simulink model "regulacja_pogodowa_model"  (R2022b)
settings: Solver=VariableStepAuto  StartTime=0.0  StopTime=tmax  MaxStep=0.2  RelTol=1e-3
values from neighbouring files (symbols this model uses):
  ap_wz = (TwpN - TzewN)/(TwewN - TzewN)    (= 3.25)    [obliczenia.m]    (also in obliczenia2.m)
  az_wz = (TwzN - TzewN)/(TwewN - TzewN)    (= 3.75)    [obliczenia.m]    (also in obliczenia2.m)
  bp_wz = (TwpN - TwewN)/(TwewN - TzewN)    (= 2.25)    [obliczenia.m]    (also in obliczenia2.m)
  bz_wz = (TwzN - TwewN)/(TwewN - TzewN)    (= 2.75)    [obliczenia.m]    (also in obliczenia2.m)
  dFmw = 0    [obliczenia.m]    (also in obliczenia2.m)
  Ki = 1    [obliczenia.m]    (also in obliczenia2.m = 0)
  Kp = 0.9*TczasRp2/(kRp2*TopuRp2)    (= 0.110974924224)    [obliczenia.m]    (also in obliczenia2.m = 1.05226274907)
  kRp = (1.3488)/0.02    (= 67.44)    [obliczenia.m]
  kRp2 = (71.1034-70)/0.02    (= 55.17)    [obliczenia.m]
  TczasRp = 10670-2648    (= 8022)    [obliczenia.m]
  TczasRp2 = 20334-TopuRp2    (= 17728)    [obliczenia.m]
  TemVec = [-20:20]    [obliczenia.m]    (also in obliczenia2.m = [-20,20])
  Ti = 3.33*TopuRp2/Kp    (= 78197.6654695)    [obliczenia.m]    (also in obliczenia2.m = 11755.1763626)
  TopN = TgpN    (= 70)    [obliczenia.m]    (also in obliczenia2.m)
  TopuRp = 2648 - 2000    (= 648)    [obliczenia.m]
  TopuRp2 = 4606 - tsok    (= 2606)    [obliczenia.m]
  Toz0 = TozN    (= 90)    [obliczenia.m]    (also in obliczenia2.m)
  TozN = TgzN    (= 90)    [obliczenia.m]    (also in obliczenia2.m)
  tsok = 2000    [obliczenia.m]    (also in obliczenia2.m = 80000)
  TwewN = 20    [obliczenia.m]    (also in obliczenia2.m)
undefined symbols (not defined in the file or in its folder): dToz
settings Model: Creator=asialalala  LastModifiedBy=asialalala
settings DataIOCC: ReturnWorkspaceOutputs=off

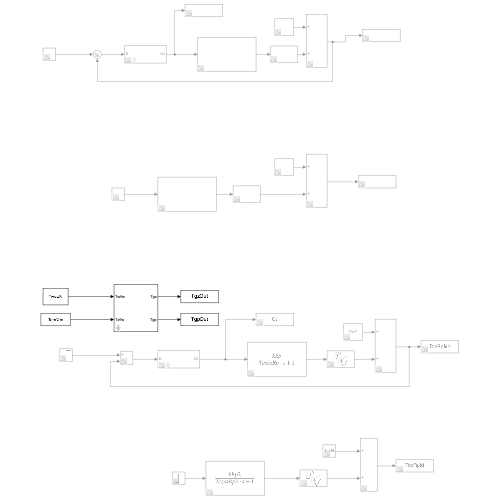
[thumbnail: Simulink's stored preview of the top-level diagram]
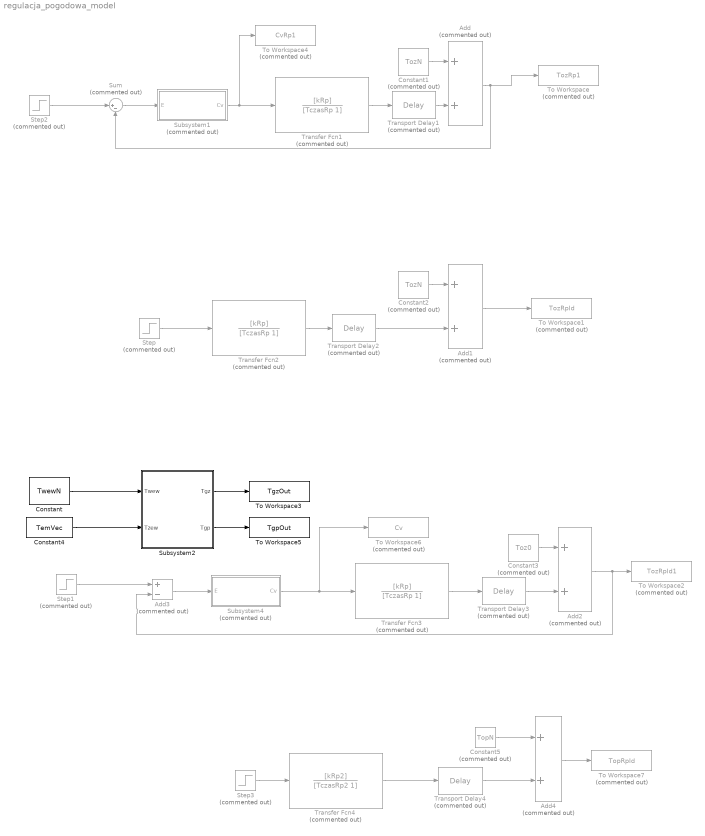
== system regulacja_pogodowa_model ==
  Add{,1..2,4} (4 alike) : Sum  Commented=on
  Add3 : Sum  Commented=on  Inputs=+-
  Constant : Constant  Value=TwewN
  Constant1 : Constant  Commented=on  Value=TozN
  Constant2 : Constant  Commented=on  Value=TozN
  Constant3 : Constant  Commented=on  Value=Toz0
  Constant4 : Constant  Value=TemVec
  Constant5 : Constant  Commented=on  Value=TopN
  Step : Step  Commented=on  Time=tsok  After=dFmw  SampleTime=0
  Step1 : Step  Commented=on  Time=tsok  Before=Toz0  After=Toz0+1  SampleTime=0
  Step2 : Step  Commented=on  Time=tsok  Before=TozN  After="TozN  + dToz"  SampleTime=0
  Step3 : Step  Commented=on  Time=tsok  After=dFmw  SampleTime=0
  Subsystem1 : Subsystem  Commented=on  mask{Kp=Kp, Ti=Ti, Cv0=0, Ki=Ki}
  Subsystem2 : Subsystem  mask{az=az_wz, bz=bz_wz, ap=ap_wz, bp=bp_wz}
  Subsystem4 : Subsystem  Commented=on  mask{Kp=Kp, Ti=Ti, Cv0=0, Ki=Ki}
  Sum : Sum  Commented=on  Inputs=|+-
  To Workspace : ToWorkspace  Commented=on  VariableName=TozRp1  SampleTime=-1
  To Workspace1 : ToWorkspace  Commented=on  VariableName=TozRpId  SampleTime=-1
  To Workspace2 : ToWorkspace  Commented=on  VariableName=TozRpId1  SampleTime=-1
  To Workspace3 : ToWorkspace  VariableName=TgzOut  SampleTime=-1
  To Workspace4 : ToWorkspace  Commented=on  VariableName=CvRp1  SampleTime=-1
  To Workspace5 : ToWorkspace  VariableName=TgpOut  SampleTime=-1
  To Workspace6 : ToWorkspace  Commented=on  VariableName=Cv  SampleTime=-1
  To Workspace7 : ToWorkspace  Commented=on  VariableName=TopRpId  SampleTime=-1
  Transfer Fcn1 : TransferFcn  Commented=on  Numerator=[kRp]  Denominator=[TczasRp 1]
  Transfer Fcn2 : TransferFcn  Commented=on  Numerator=[kRp]  Denominator=[TczasRp 1]
  Transfer Fcn3 : TransferFcn  Commented=on  Numerator=[kRp]  Denominator=[TczasRp 1]
  Transfer Fcn4 : TransferFcn  Commented=on  Numerator=[kRp2]  Denominator=[TczasRp2 1]
  Transport Delay1 : TransportDelay  Commented=on  DelayTime=TopuRp
  Transport Delay2 : TransportDelay  Commented=on  DelayTime=TopuRp
  Transport Delay3 : TransportDelay  Commented=on  DelayTime=TopuRp
  Transport Delay4 : TransportDelay  Commented=on  DelayTime=TopuRp2
  wires:
  Add/1 -> Sum/2, To Workspace/1
  Constant1/1 -> Add/1
  Step2/1 -> Sum/1
  Subsystem1/1(Cv) -> To Workspace4/1, Transfer Fcn1/1
  Transfer Fcn1/1 -> Transport Delay1/1
  Transport Delay1/1 -> Add/2
  Sum/1 -> Subsystem1/1(E)
  Step/1 -> Transfer Fcn2/1
  Transfer Fcn2/1 -> Transport Delay2/1
  Transport Delay2/1 -> Add1/2
  Add1/1 -> To Workspace1/1
  Constant2/1 -> Add1/1
  Transfer Fcn3/1 -> Transport Delay3/1
  Transport Delay3/1 -> Add2/2
  Constant3/1 -> Add2/1
  Add2/1 -> Add3/2, To Workspace2/1
  Constant/1 -> Subsystem2/1(Twew)
  Constant4/1 -> Subsystem2/2(Tzew)
  Subsystem2/1(Tgz) -> To Workspace3/1
  Subsystem2/2(Tgp) -> To Workspace5/1
  Add3/1 -> Subsystem4/1(E)
  Subsystem4/1(Cv) -> To Workspace6/1, Transfer Fcn3/1
  Step1/1 -> Add3/1
  Step3/1 -> Transfer Fcn4/1
  Transfer Fcn4/1 -> Transport Delay4/1
  Add4/1 -> To Workspace7/1
  Constant5/1 -> Add4/1
  Transport Delay4/1 -> Add4/2

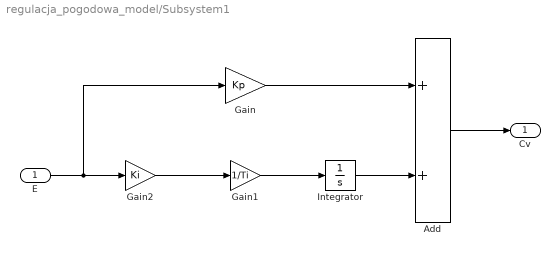
== system regulacja_pogodowa_model/Subsystem1 ==
  E : Inport
  Add : Sum
  Gain : Gain  Gain=Kp
  Gain1 : Gain  Gain=1/Ti
  Gain2 : Gain  Gain=Ki
  Integrator : Integrator  InitialCondition=Cv0
  Cv : Outport
  wires:
  E/1 -> Gain/1, Gain2/1
  Gain2/1 -> Gain1/1
  Gain1/1 -> Integrator/1
  Add/1 -> Cv/1
  Gain/1 -> Add/1
  Integrator/1 -> Add/2

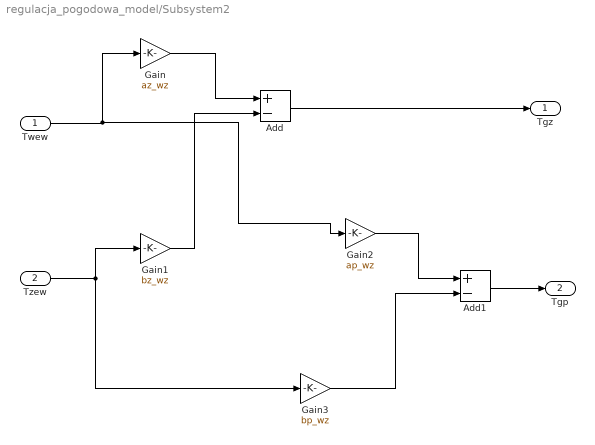
== system regulacja_pogodowa_model/Subsystem2 ==
  Twew : Inport
  Tzew : Inport  Port=2
  Add : Sum  Inputs=+-
  Add1 : Sum  Inputs=+-
  Gain : Gain  Gain=az_wz
  Gain1 : Gain  Gain=bz_wz
  Gain2 : Gain  Gain=ap_wz
  Gain3 : Gain  Gain=bp_wz
  Tgz : Outport
  Tgp : Outport  Port=2
  wires:
  Gain1/1 -> Add/2
  Gain/1 -> Add/1
  Add/1 -> Tgz/1
  Add1/1 -> Tgp/1
  Twew/1 -> Gain2/1, Gain/1
  Gain2/1 -> Add1/1
  Tzew/1 -> Gain3/1, Gain1/1
  Gain3/1 -> Add1/2

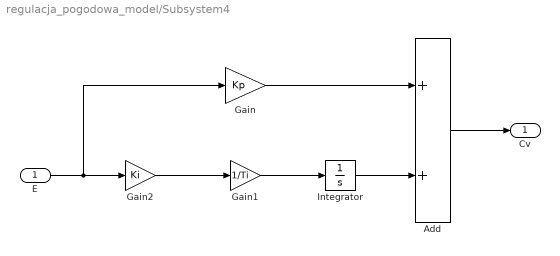
== system regulacja_pogodowa_model/Subsystem4 ==
  E : Inport
  Add : Sum
  Gain : Gain  Gain=Kp
  Gain1 : Gain  Gain=1/Ti
  Gain2 : Gain  Gain=Ki
  Integrator : Integrator  InitialCondition=Cv0
  Cv : Outport
  wires:
  E/1 -> Gain/1, Gain2/1
  Gain2/1 -> Gain1/1
  Gain1/1 -> Integrator/1
  Add/1 -> Cv/1
  Gain/1 -> Add/1
  Integrator/1 -> Add/2
